simulink model "Simulator"  (R2016b)
settings: Solver=VariableStepAuto  StartTime=0.0  StopTime=simulation_time  RelTol=1e-3  EnableMultiTasking=on
InitFcn:
  | Parameters_quadrotor
undefined symbols (not defined in the file or in its folder): delay_attitude, delay_mixer, delay_position, dLMN, gravity, inertia_tensor, inertia_tensor_inv, K, magnitude, mass, mass_matrix, mass_matrix_inv, motor_ome_vs_throttle, motor_tau, sample_time, sigbuilder_block
libraries: aerolibutil x2
settings Model: Creator=Mattia  LastModifiedBy=Mattia
settings DataIOCC: SaveFormat=Array
settings OptimizationCC: LifeSpan=inf
settings DebuggingCC: SFUnexpectedBacktrackingDiag=warning  SFNoUnconditionalDefaultTransitionDiag=warning  SFExecutionAtInitializationDiag=none
settings GRTTargetCC: TargetLangStandard=C89/C90 (ANSI)  GeneratePreprocessorConditionals=Disable all
settings ConfigComp: CovMetricSettings=dw  CovHtmlReporting=on  CovSaveCumulativeToWorkspaceVar=on  CovSaveSingleToWorkspaceVar=on  CovExternalEMLEnable=off

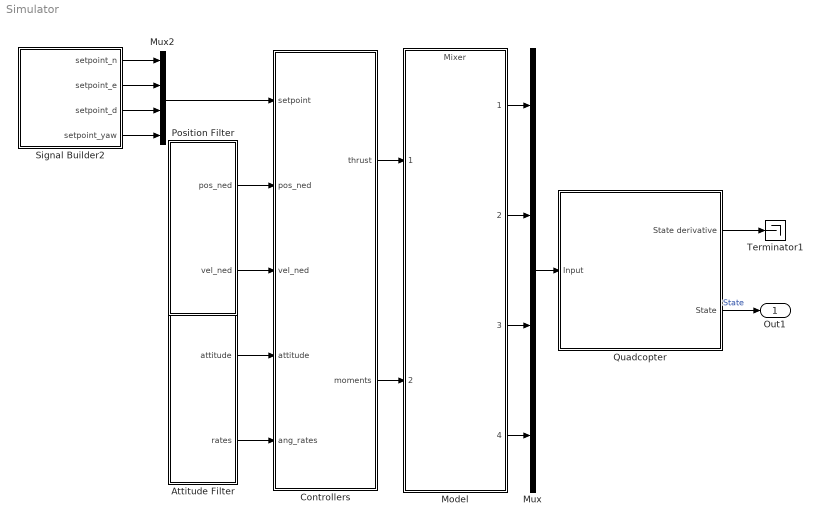
== system Simulator ==
  Attitude Filter : Subsystem
  Controllers : Subsystem
  Model : ModelReference  ModelNameDialog=Mixer.slx  SimulationMode=Normal  ModelReferenceVersion=1.35
  Mux : Mux
  Mux2 : Mux
  Position Filter : Subsystem
  Quadcopter : Subsystem
      mask Display:
      | image(imread('quad.png'))
      | port_label('input',1,'u')
      | port_label('output',1,'Xdot')
      | port_label('output',2,'X')
  Signal Builder2 : Subsystem  Tag=STV Subsys  LoadFcn=sigbuilder_block('load');  StartFcn=sigbuilder_block('start');  StopFcn=sigbuilder_block('stop');  ClipboardFcn=sigbuilder_block('clipboard');  mask(Sigbuilder block){tuvar=[0:10]}
      mask help: Simulink:masks:SigbuilderBlock_MD
      mask init:
      | if ~strcmp(get_param(bdroot(gcbh),'SimulationStatus'),'stopped') tuvar = sigbuilder_block('maskInit'); end
      settings: CopyFcn=sigbuilder_block('copy');  DeleteFcn=sigbuilder_block('delete');  ModelCloseFcn=sigbuilder_block('modelClose');  PreSaveFcn=sigbuilder_block('preSave');  PauseFcn=sigbuilder_block('pause');  ContinueFcn=sigbuilder_block('continue');  NameChangeFcn=sigbuilder_block('namechange');  OpenFcn=sigbuilder_block('open',[0 30 1024.5 488.25 ]);  CloseFcn=sigbuilder_block('close');
      mask Display: plot(0, 0, 100, 100,[2, 2, 32, 32, 2], [68, 8, 8, 68, 68],[32, 2], [38, 38], [32, 19, 2],[53, 60, 44], [32, 17, 17, 2],[16, 16, 31, 31]);txt = getActiveGroup(gcbh);text(2, 100, txt,'verticalAlignment', 'top');
  Terminator1 : Terminator
  Out1 : Outport
  wires:
  Signal Builder2/2(setpoint_e) -> Mux2/2
  Signal Builder2/3(setpoint_d) -> Mux2/3
  Signal Builder2/4("setpoint_yaw ") -> Mux2/4
  Signal Builder2/1(setpoint_n) -> Mux2/1
  Controllers/2(moments) -> Model/2
  Mux2/1 -> Controllers/1(setpoint)
  Quadcopter/1(State derivative) -> Terminator1/1
  Attitude Filter/1(attitude) -> Controllers/4(attitude)
  Mux/1 -> Quadcopter/1(Input)
  Model/1 -> Mux/1
  Model/2 -> Mux/2
  Model/3 -> Mux/3
  Model/4 -> Mux/4
  Controllers/1(thrust) -> Model/1
  Attitude Filter/2(rates) -> Controllers/5(ang_rates)
  Position Filter/1(pos_ned) -> Controllers/2(pos_ned)
  Position Filter/2(vel_ned) -> Controllers/3(vel_ned)
  Quadcopter/2(State) -> Out1/1  "State"

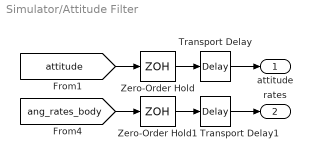
== system Simulator/Attitude Filter ==
  Transport Delay : TransportDelay  DelayTime=delay_attitude * sample_time
  Transport Delay1 : TransportDelay  DelayTime=delay_attitude * sample_time
  Zero-Order Hold : ZeroOrderHold  SampleTime=sample_time
  Zero-Order Hold1 : ZeroOrderHold  SampleTime=sample_time
  attitude : Outport  PortDimensions=3
  rates : Outport  Port=2  PortDimensions=3
  wires:
  [ang_rates_body] -> Zero-Order Hold1/1
  [attitude] -> Zero-Order Hold/1
  Zero-Order Hold1/1 -> Transport Delay1/1
  Zero-Order Hold/1 -> Transport Delay/1
  Transport Delay1/1 -> rates/1
  Transport Delay/1 -> attitude/1

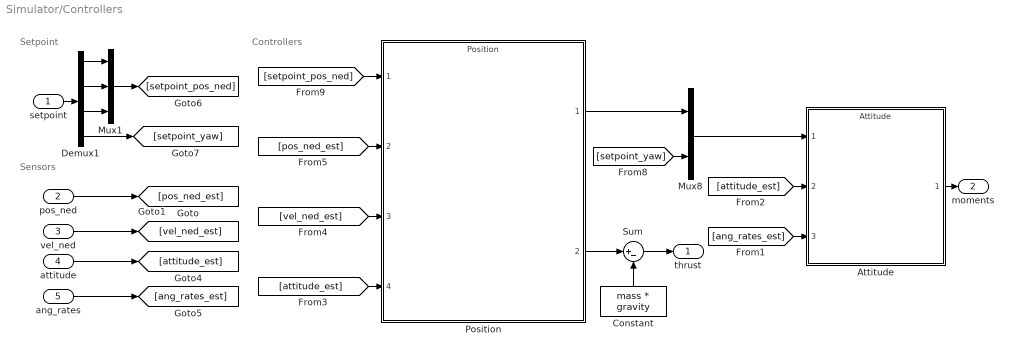
== system Simulator/Controllers ==
  note: Sensors
  note: Setpoint
  note: Controllers
  setpoint : Inport  PortDimensions=4
  pos_ned : Inport  Port=2  PortDimensions=3
  vel_ned : Inport  Port=3  PortDimensions=3
  attitude : Inport  Port=4  PortDimensions=3
  ang_rates : Inport  Port=5  PortDimensions=3
  Attitude : ModelReference  ModelNameDialog=Attitude.slx  SimulationMode=Normal  ModelReferenceVersion=1.162
  Constant : Constant  Value=mass * gravity
  Demux1 : Demux
  Mux1 : Mux  Inputs=3
  Mux8 : Mux  Inputs=2
  Position : ModelReference  ModelNameDialog=Position.slx  SimulationMode=Normal  ModelReferenceVersion=1.303
  Sum : Sum  Inputs=|+-
  thrust : Outport
  moments : Outport  Port=2  PortDimensions=3
  wires:
  setpoint/1 -> Demux1/1
  [attitude_est] -> Attitude/2
  Demux1/4 -> [setpoint_yaw]
  Demux1/2 -> Mux1/2
  Demux1/1 -> Mux1/1
  Attitude/1 -> moments/1
  [pos_ned_est] -> Position/2
  Mux8/1 -> Attitude/1
  [ang_rates_est] -> Attitude/3
  Constant/1 -> Sum/2
  [setpoint_yaw] -> Mux8/2
  attitude/1 -> [attitude_est]
  Mux1/1 -> [setpoint_pos_ned]
  [setpoint_pos_ned] -> Position/1
  pos_ned/1 -> [pos_ned_est]
  vel_ned/1 -> [vel_ned_est]
  ang_rates/1 -> [ang_rates_est]
  [attitude_est] -> Position/4
  Sum/1 -> thrust/1
  [vel_ned_est] -> Position/3
  Demux1/3 -> Mux1/3
  Position/1 -> Mux8/1
  Position/2 -> Sum/1

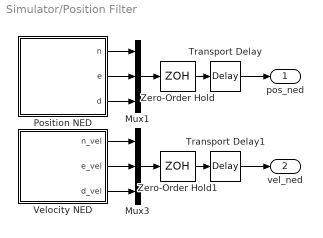
== system Simulator/Position Filter ==
  Mux1 : Mux  Inputs=3
  Mux3 : Mux  Inputs=3
  Position NED : Subsystem
  Transport Delay : TransportDelay  DelayTime=delay_position * sample_time
  Transport Delay1 : TransportDelay  DelayTime=delay_position * sample_time
  Velocity NED : Subsystem
  Zero-Order Hold : ZeroOrderHold  SampleTime=sample_time
  Zero-Order Hold1 : ZeroOrderHold  SampleTime=sample_time
  pos_ned : Outport  PortDimensions=3
  vel_ned : Outport  Port=2  PortDimensions=3
  wires:
  Position NED/2(e) -> Mux1/2
  Velocity NED/2(e_vel) -> Mux3/2
  Velocity NED/1(n_vel) -> Mux3/1
  Position NED/1(n) -> Mux1/1
  Zero-Order Hold/1 -> Transport Delay/1
  Mux1/1 -> Zero-Order Hold/1
  Transport Delay/1 -> pos_ned/1
  Zero-Order Hold1/1 -> Transport Delay1/1
  Mux3/1 -> Zero-Order Hold1/1
  Transport Delay1/1 -> vel_ned/1
  Position NED/3(d) -> Mux1/3
  Velocity NED/3(d_vel) -> Mux3/3

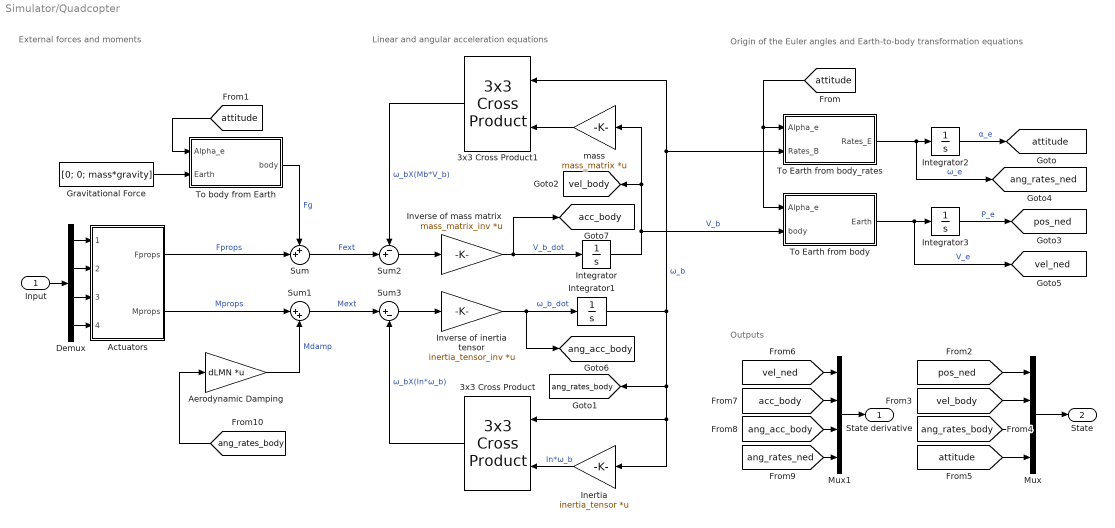
== system Simulator/Quadcopter ==
  note: Outputs
  note: Origin of the Euler angles and Earth-to-body transformation equations
  note: Linear and angular acceleration equations
  note: External forces and moments
  Input : Inport
  3x3 Cross Product : aerolibutil/3x3 Cross Product
  3x3 Cross Product1 : aerolibutil/3x3 Cross Product
  Actuators : Subsystem
  Aerodynamic Damping : Gain  Gain=dLMN  Multiplication=Matrix(K*u)
  Demux : Demux
  Gravitational Force : Constant  Value=[0; 0; mass*gravity]
  Inertia : Gain  Gain=inertia_tensor  Multiplication=Matrix(K*u)
  Integrator{,1..3} (4 alike) : Integrator  InitialCondition=[0; 0; 0]
  Inverse of inertia tensor : Gain  Gain=inertia_tensor_inv  Multiplication=Matrix(K*u)
  Inverse of mass matrix : Gain  Gain=mass_matrix_inv  Multiplication=Matrix(K*u)
  Mux : Mux
  Mux1 : Mux
  Sum : Sum  Inputs=++|
  Sum1 : Sum  Inputs=|++
  Sum2 : Sum  Inputs=-+|
  Sum3 : Sum  Inputs=|+-
  To Earth from body : MATLAB Function  TreatAsAtomicUnit=on
  To Earth from body_rates : MATLAB Function  TreatAsAtomicUnit=on
  To body from Earth : MATLAB Function  TreatAsAtomicUnit=on
  mass : Gain  Gain=mass_matrix  Multiplication=Matrix(K*u)
  State derivative : Outport
  State : Outport  Port=2
  tag scope: acc_body=global, ang_acc_body=global, ang_rates_body=global, ang_rates_ned=global, attitude=global, pos_ned=global, vel_body=global, vel_ned=global
  wires:
  To Earth from body_rates/1(Rates_E) -> Integrator2/1, [ang_rates_ned]  "ω_e"
  [pos_ned] -> Mux/1
  Actuators/2(Mprops) -> Sum1/1  "Mprops"
  Input/1 -> Demux/1
  3x3 Cross Product/1 -> Sum3/2  "ω_bX(In*ω_b)"
  [acc_body] -> Mux1/2
  Mux/1 -> State/1
  Mux1/1 -> State derivative/1
  [vel_body] -> Mux/2
  [attitude] -> Mux/4
  [ang_rates_body] -> Mux/3
  Demux/4 -> Actuators/4(Th4 [%])
  [ang_rates_ned] -> Mux1/4
  [ang_acc_body] -> Mux1/3
  [vel_ned] -> Mux1/1
  Demux/3 -> Actuators/3(Th3 [%])
  Inverse of mass matrix/1 -> Integrator/1, [acc_body]  "V_b_dot"
  Integrator/1 -> To Earth from body/2(body), mass/1, [vel_body]  "V_b"
  [attitude] -> To Earth from body/1(Alpha_e), To Earth from body_rates/1(Alpha_e)
  Integrator1/1 -> To Earth from body_rates/2(Rates_B), 3x3 Cross Product1/1, 3x3 Cross Product/1, Inertia/1, [ang_rates_body]  "ω_b"
  Sum3/1 -> Inverse of inertia tensor/1
  Sum2/1 -> Inverse of mass matrix/1
  mass/1 -> 3x3 Cross Product1/2
  Sum/1 -> Sum2/2  "Fext"
  Sum1/1 -> Sum3/1  "Mext"
  Demux/1 -> Actuators/1(Th1 [%])
  Demux/2 -> Actuators/2(Th2 [%])
  Inverse of inertia tensor/1 -> Integrator1/1, [ang_acc_body]  "ω_b_dot"
  3x3 Cross Product1/1 -> Sum2/1  "ω_bX(Mb*V_b)"
  Integrator2/1 -> [attitude]  "α_e"
  Aerodynamic Damping/1 -> Sum1/2  "Mdamp"
  Actuators/1(Fprops) -> Sum/2  "Fprops"
  Integrator3/1 -> [pos_ned]  "P_e"
  Inertia/1 -> 3x3 Cross Product/2  "In*ω_b"
  [ang_rates_body] -> Aerodynamic Damping/1
  To Earth from body/1(Earth) -> [vel_ned], Integrator3/1  "V_e"
  To body from Earth/1(body) -> Sum/1  "Fg"
  Gravitational Force/1 -> To body from Earth/2(Earth)
  [attitude] -> To body from Earth/1(Alpha_e)

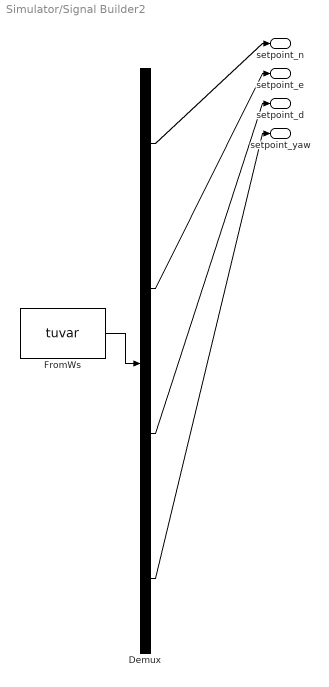
== system Simulator/Signal Builder2 ==
  Demux : Demux  Tag=STV Demux
  FromWs : FromWorkspace  Tag=STV FromWs  VariableName=tuvar  SampleTime=0
      SigBuilderData=|
      | common.afterFinalStr = 'Extrapolate'
      | common.sampleTime = 0
      | dataSet(1).timeRange = [0 50]
      | dataSet(1).name = 'setpoint'
      | dataSet(2).timeRange = [0 50]
      | dataSet(2).name = 'Set-point_2'
      | sbobj.Groups(1).Name = 'setpoint'
      | sbobj.Groups(1).Signals(1).Name = 'setpoint_n'
      | sbobj.Groups(1).Signals(1).XData = [0 10 13 30 33 50]
      | sbobj.Groups(1).Signals(1).YData = [0 0 1 1 0 0]
      | sbobj.Groups(1).Signals(2).Name = 'setpoint_e'
      | sbobj.Groups(1).Signals(2).XData = [0 50]
      | sbobj.Groups(1).Signals(2).YData = [0 0]
      | sbobj.Groups(1).Signals(3).Name = 'setpoint_d'
      | sbobj.Groups(1).Signals(3).XData = [0 50]
      | sbobj.Groups(1).Signals(3).YData = [-1 -1]
      | sbobj.Groups(1).Signals(4).Name = 'setpoint_yaw '
      | sbobj.Groups(1).Signals(4).XData = [0 10 40 50]
      | sbobj.Groups(1).Signals(4).YData = [0 0 0 0]
      | sbobj.Groups(1).TimeRange = [0 50]
      | sbobj.Groups(2).Name = 'Set-point_2'
      | sbobj.Groups(2).Signals(1).Name = 'setpoint_n'
      | sbobj.Groups(2).Signals(1).XData = [0 10 45 45.05 50]
      | sbobj.Groups(2).Signals(1).YData = [0 0 1 0 0]
      | sbobj.Groups(2).Signals(2).Name = 'setpoint_e'
      | sbobj.Groups(2).Signals(2).XData = [0 10 50]
      | sbobj.Groups(2).Signals(2).YData = [0 0 0]
      | sbobj.Groups(2).Signals(3).Name = 'setpoint_d'
      | sbobj.Groups(2).Signals(3).XData = [0 50]
      | sbobj.Groups(2).Signals(3).YData = [-2 -2]
      | sbobj.Groups(2).Signals(4).Name = 'setpoint_yaw '
      | sbobj.Groups(2).Signals(4).XData = [0 10 40 50]
      | sbobj.Groups(2).Signals(4).YData = [0 0 0 0]
      | sbobj.Groups(2).TimeRange = [0 50]
  setpoint_n : Outport  Tag=STV Outport
  setpoint_e : Outport  Tag=STV Outport  Port=2
  setpoint_d : Outport  Tag=STV Outport  Port=3
  "setpoint_yaw " : Outport  Tag=STV Outport  Port=4
  wires:
  FromWs/1 -> Demux/1
  Demux/1 -> setpoint_n/1
  Demux/2 -> setpoint_e/1
  Demux/3 -> setpoint_d/1
  Demux/4 -> "setpoint_yaw "/1

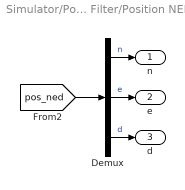
== system Simulator/Position Filter/Position NED ==
  Demux : Demux  Outputs=3
  n : Outport
  e : Outport  Port=2
  d : Outport  Port=3
  wires:
  Demux/1 -> n/1  "n"
  Demux/3 -> d/1  "d"
  [pos_ned] -> Demux/1
  Demux/2 -> e/1  "e"

== system Simulator/Position Filter/Velocity NED ==
  Demux : Demux  Outputs=3
  n_vel : Outport
  e_vel : Outport  Port=2
  d_vel : Outport  Port=3
  wires:
  Demux/2 -> e_vel/1  "e"
  [vel_ned] -> Demux/1
  Demux/3 -> d_vel/1  "d"
  Demux/1 -> n_vel/1  "n"

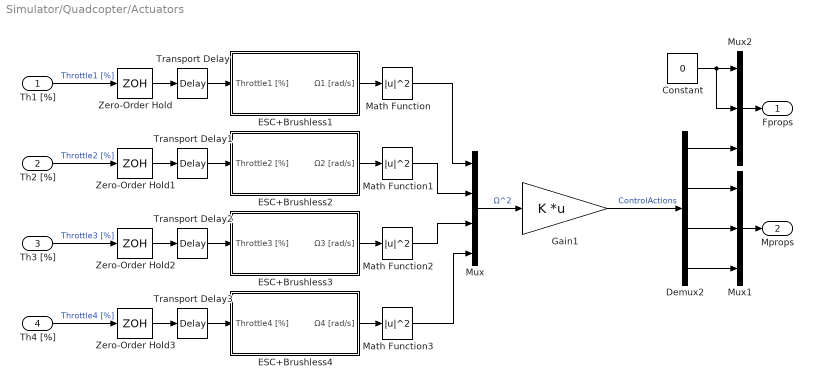
== system Simulator/Quadcopter/Actuators ==
  Th1 [%] : Inport
  Th2 [%] : Inport  Port=2
  Th3 [%] : Inport  Port=3
  Th4 [%] : Inport  Port=4
  Constant : Constant  Value=0
  Demux2 : Demux
  ESC+Brushless1 : Subsystem
  ESC+Brushless2 : Subsystem
  ESC+Brushless3 : Subsystem
  ESC+Brushless4 : Subsystem
  Gain1 : Gain  Gain=K  Multiplication=Matrix(K*u)
  Math Function{,1..3} (4 alike) : Math  Operator=magnitude^2  SaturateOnIntegerOverflow=on
  Mux : Mux
  Mux1 : Mux  Inputs=3
  Mux2 : Mux  Inputs=3
  Transport Delay{,1..3} (4 alike) : TransportDelay  DelayTime=delay_mixer * sample_time
  Zero-Order Hold{,1..3} (4 alike) : ZeroOrderHold  SampleTime=sample_time
  Fprops : Outport
  Mprops : Outport  Port=2
  wires:
  Gain1/1 -> Demux2/1  "ControlActions"
  Th1 [%]/1 -> Zero-Order Hold/1  "Throttle1 [%]"
  Th2 [%]/1 -> Zero-Order Hold1/1  "Throttle2 [%]"
  Th4 [%]/1 -> Zero-Order Hold3/1  "Throttle4 [%]"
  Th3 [%]/1 -> Zero-Order Hold2/1  "Throttle3 [%]"
  ESC+Brushless1/1(Ω1 [rad/s]) -> Math Function/1
  ESC+Brushless2/1(Ω2 [rad/s]) -> Math Function1/1
  ESC+Brushless3/1(Ω3 [rad/s]) -> Math Function2/1
  ESC+Brushless4/1(Ω4 [rad/s]) -> Math Function3/1
  Mux/1 -> Gain1/1  "Ω^2"
  Math Function/1 -> Mux/1
  Math Function1/1 -> Mux/2
  Math Function2/1 -> Mux/3
  Math Function3/1 -> Mux/4
  Mux1/1 -> Mprops/1
  Demux2/2 -> Mux1/1
  Demux2/3 -> Mux1/2
  Demux2/4 -> Mux1/3
  Demux2/1 -> Mux2/3
  Constant/1 -> Mux2/2, Mux2/1
  Mux2/1 -> Fprops/1
  Transport Delay/1 -> ESC+Brushless1/1(Throttle1 [%])
  Transport Delay1/1 -> ESC+Brushless2/1(Throttle2 [%])
  Transport Delay3/1 -> ESC+Brushless4/1(Throttle4 [%])
  Transport Delay2/1 -> ESC+Brushless3/1(Throttle3 [%])
  Zero-Order Hold/1 -> Transport Delay/1
  Zero-Order Hold1/1 -> Transport Delay1/1
  Zero-Order Hold2/1 -> Transport Delay2/1
  Zero-Order Hold3/1 -> Transport Delay3/1

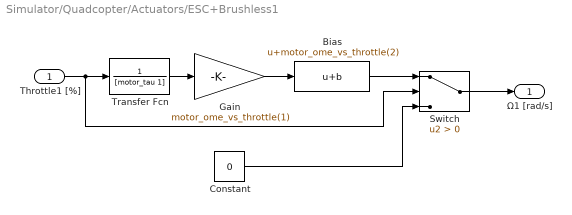
== system Simulator/Quadcopter/Actuators/ESC+Brushless1 ==
  Throttle1 [%] : Inport
  Bias : Bias  Bias=motor_ome_vs_throttle(2)
  Constant : Constant  Value=0
  Gain : Gain  Gain=motor_ome_vs_throttle(1)
  Switch : Switch  Criteria=u2 > Threshold
  Transfer Fcn : TransferFcn  Denominator=[motor_tau 1]
  Ω1 [rad/s] : Outport
  wires:
  Gain/1 -> Bias/1
  Bias/1 -> Switch/1
  Constant/1 -> Switch/3
  Switch/1 -> Ω1 [rad/s]/1
  Throttle1 [%]/1 -> Transfer Fcn/1, Switch/2
  Transfer Fcn/1 -> Gain/1

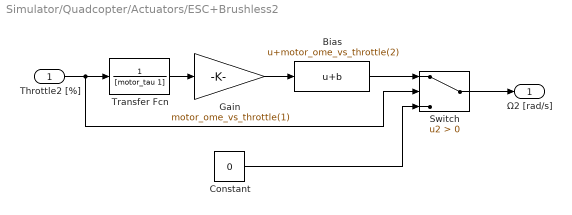
== system Simulator/Quadcopter/Actuators/ESC+Brushless2 ==
  Throttle2 [%] : Inport
  Bias : Bias  Bias=motor_ome_vs_throttle(2)
  Constant : Constant  Value=0
  Gain : Gain  Gain=motor_ome_vs_throttle(1)
  Switch : Switch  Criteria=u2 > Threshold
  Transfer Fcn : TransferFcn  Denominator=[motor_tau 1]
  Ω2 [rad/s] : Outport
  wires:
  Gain/1 -> Bias/1
  Bias/1 -> Switch/1
  Constant/1 -> Switch/3
  Switch/1 -> Ω2 [rad/s]/1
  Throttle2 [%]/1 -> Transfer Fcn/1, Switch/2
  Transfer Fcn/1 -> Gain/1

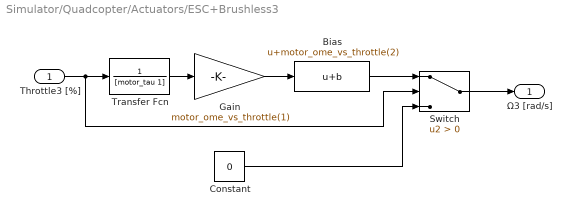
== system Simulator/Quadcopter/Actuators/ESC+Brushless3 ==
  Throttle3 [%] : Inport
  Bias : Bias  Bias=motor_ome_vs_throttle(2)
  Constant : Constant  Value=0
  Gain : Gain  Gain=motor_ome_vs_throttle(1)
  Switch : Switch  Criteria=u2 > Threshold
  Transfer Fcn : TransferFcn  Denominator=[motor_tau 1]
  Ω3 [rad/s] : Outport
  wires:
  Gain/1 -> Bias/1
  Bias/1 -> Switch/1
  Constant/1 -> Switch/3
  Switch/1 -> Ω3 [rad/s]/1
  Throttle3 [%]/1 -> Transfer Fcn/1, Switch/2
  Transfer Fcn/1 -> Gain/1

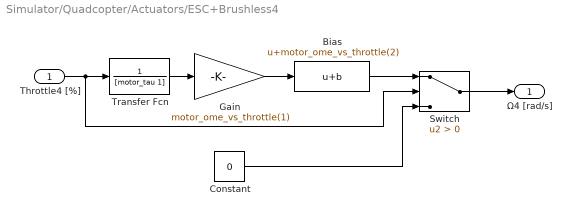
== system Simulator/Quadcopter/Actuators/ESC+Brushless4 ==
  Throttle4 [%] : Inport
  Bias : Bias  Bias=motor_ome_vs_throttle(2)
  Constant : Constant  Value=0
  Gain : Gain  Gain=motor_ome_vs_throttle(1)
  Switch : Switch  Criteria=u2 > Threshold
  Transfer Fcn : TransferFcn  Denominator=[motor_tau 1]
  Ω4 [rad/s] : Outport
  wires:
  Gain/1 -> Bias/1
  Bias/1 -> Switch/1
  Constant/1 -> Switch/3
  Switch/1 -> Ω4 [rad/s]/1
  Throttle4 [%]/1 -> Transfer Fcn/1, Switch/2
  Transfer Fcn/1 -> Gain/1

== matlab function Simulator/Quadcopter/To body from Earth ==
  data: Alpha_e input; Earth input; body output
 function body = Tbe(Alpha_e, Earth)
%#codegen
phi = Alpha_e(1);
theta = Alpha_e(2);
psi = Alpha_e(3);

Sphi = sin(phi);
Cphi = cos(phi);
Stheta = sin(theta);
Ctheta = cos(theta);
Spsi = sin(psi);
Cpsi = cos(psi);

TBE = [        Ctheta*Cpsi               Ctheta*Spsi          -Stheta    ;
       Sphi*Stheta*Cpsi-Cphi*Spsi Sphi*Stheta*Spsi+Cphi*Cpsi Sphi*Ctheta ;
       Cphi*Stheta*Cpsi+Sphi*Spsi Cphi*Stheta*Spsi-Sphi*Cpsi Cphi*Ctheta];

body = TBE* Earth;

== matlab function Simulator/Quadcopter/To Earth from body ==
  data: Alpha_e input; Earth output; body input
 function Earth = Tbet(Alpha_e, body)
%#codegen
phi = Alpha_e(1);
theta = Alpha_e(2);
psi = Alpha_e(3);

Sphi = sin(phi);
Cphi = cos(phi);
Stheta = sin(theta);
Ctheta = cos(theta);
Spsi = sin(psi);
Cpsi = cos(psi);

TBE = [        Ctheta*Cpsi               Ctheta*Spsi          -Stheta    ;
       Sphi*Stheta*Cpsi-Cphi*Spsi Sphi*Stheta*Spsi+Cphi*Cpsi Sphi*Ctheta ;
       Cphi*Stheta*Cpsi+Sphi*Spsi Cphi*Stheta*Spsi-Sphi*Cpsi Cphi*Ctheta];
TEB = TBE';

Earth = TEB* body;

== matlab function Simulator/Quadcopter/To Earth from body_rates ==
  data: Alpha_e input; Rates_B input; Rates_E output
 function Rates_E = Einv(Alpha_e, Rates_B)
%#codegen
phi = Alpha_e(1);
theta = Alpha_e(2);

Sphi = sin(phi);
Cphi = cos(phi);
Ctheta = cos(theta);
Ttheta = tan(theta);

Einv = [1   Sphi*Ttheta    Cphi*Ttheta ;
        0       Cphi          -Sphi    ;
        0   Sphi/Ctheta    Cphi/Ctheta];

Rates_E = Einv* Rates_B;
